simulink model "RegulatedBuckConverter"  (R2021b)
settings: Solver=ode23tb  StartTime=0.0  StopTime=0.5  RelTol=1e-4  EnableMultiTasking=on
PreLoadFcn:
  | Ts=10e-6;
InitFcn:
  | Ts=10e-6;
libraries: spsGroundLib x3, spsDCVoltageSourceLib x2, spsBuckConverterLib x1, spsDCMachineLib x1, spsFirstOrderFilterLib x1, spsSeriesRLCBranchLib x1, spsMeanLib x1, spsVoltageMeasurementLib x1, spspowerguiLib x1
settings Model: Creator=The MathWorks, Inc.  LastModifiedBy=francescobazzani
settings SolverCC: AlgebraicLoopSolver=TrustRegion  SolverResetMethod=Robust
settings DataIOCC: SaveFormat=StructureWithTime  SaveOutput=off  SignalLogging=off  DSMLogging=off  VisualizeSimOutput=off  SaveTime=off  ReturnWorkspaceOutputs=off
settings OptimizationCC: LifeSpan=inf
settings DebuggingCC: UnconnectedInputMsg=none  UnconnectedOutputMsg=none  UnconnectedLineMsg=none  AllowSymbolicDim=off  SFUnexpectedBacktrackingDiag=warning  SFNoUnconditionalDefaultTransitionDiag=warning  SFExecutionAtInitializationDiag=none  SFMachineParentedDataDiag=warning  ArithmeticOperatorsInVariantConditions=warning
settings ModelReferenceCC: PropagateSignalLabelsOutOfModel=off
settings SFSimCC: SimUseLocalCustomCode=off  CustomCodeUndefinedFunction=UseInterfaceOnly
settings RTWCC: RTWUseLocalCustomCode=off
settings CodeAppCC: StateflowObjectComments=on
settings GRTTargetCC: TargetLangStandard=C89/C90 (ANSI)
settings ConfigComp: CovMetricSettings=dw  CovSaveCumulativeToWorkspaceVar=on  CovSaveSingleToWorkspaceVar=on  CovExternalEMLEnable=off
settings SimscapeCC: SimscapeNormalizeSystem=off  SimscapeNominalValues={1, 'bar'; 1, 'cm^3/s'; 1, 'bar*kg/s'; 1, 'kJ/kg'; 1, 'kW'; }

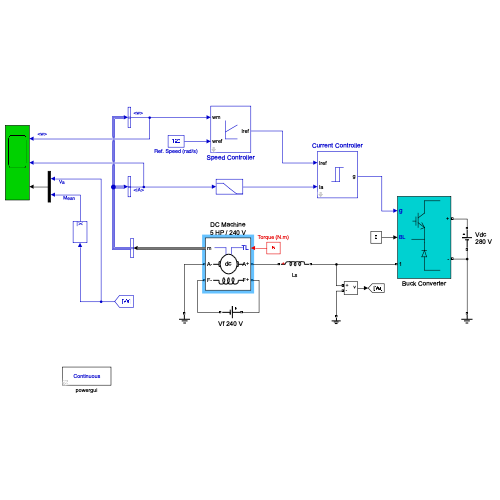
[thumbnail: Simulink's stored preview of the top-level diagram]
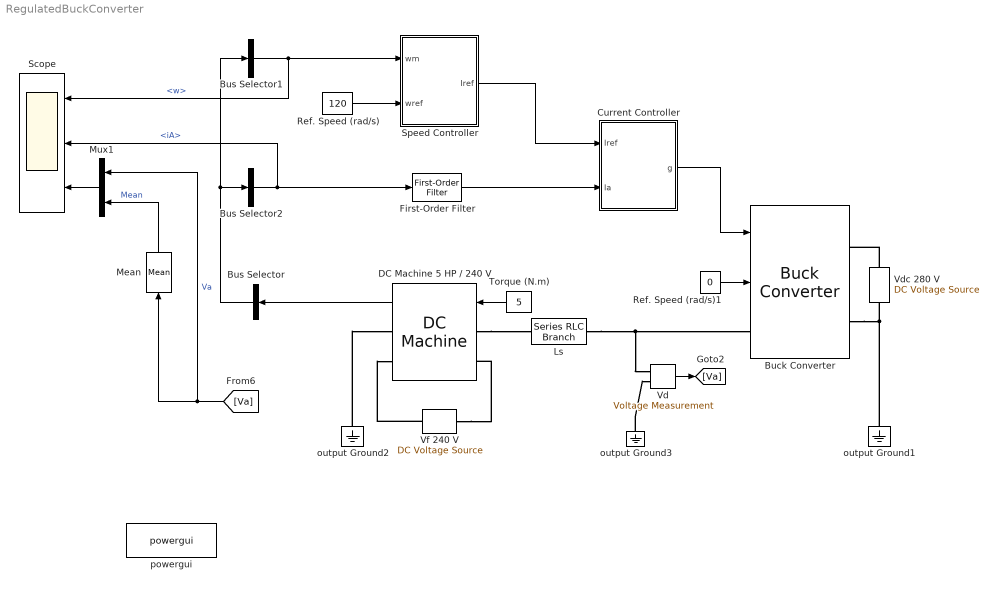
== system RegulatedBuckConverter ==
  Buck Converter : spsBuckConverterLib/Buck Converter  ModelType=Switching devices  Ron=1e-3  Rs=1e6  Cs=inf  Vforward=[0,0]  Ron_Diode=1e-3  Rs_Diode=1e6  Cs_Diode=inf  Vf_Diode=1e-3  Rs_CurrentSource=inf
      settings: SourceProductBaseCode=PS
  Bus Selector : BusSelector  OutputSignals=w,iA  OutputAsBus=on
  Bus Selector1 : BusSelector  OutputSignals=w
  Bus Selector2 : BusSelector  OutputSignals=iA
  Current Controller : Subsystem  mask{h=2}
      mask prompts: h "Hysteresis band (A)"
      mask help: Hysteresis Current Controller
      mask Display: plot(0,0,100,100,[45,45],[35,65],[55,55],[35,65],[45,65],[65,65],[35,55],[35,35])
  DC Machine 5 HP / 240 V : spsDCMachineLib/DC Machine  PresetModel=No  MechanicalLoad=Torque TL  FieldType=Wound  ShowDetailedParameters=on  MeasurementBus=on  RLa="[ 0.5  0.01]"  RLf="[ 240  120]"  Laf=1.23  MachineConstant=Torque constant (N.m/A)  Ke=1.8  Kt=1.8  J=0.05  Bm=0.02  Tf=0  w0=0  Ifinit=1  TsPowergui=0  TsBlock=-1
  First-Order Filter : spsFirstOrderFilterLib/First-Order Filter  FilterType=Lowpass  Tc=10e-6  Ts=0  Initialize=off  Vac_Init=[0, 0, 60]  Vdc_Init=0  PlotResponse=off  FreqRange="[0,  200,  1]"
  Ls : spsSeriesRLCBranchLib/Series RLC Branch  LConnTagsString=__new0  RConnTagsString=__new0  BranchType=L  Resistance=0.01  Inductance=10e-3  SetiL0=off  InitialCurrent=30  Capacitance=[]  Setx0=off  InitialVoltage=0  Measurements=None
  Mean : spsMeanLib/Mean  Freq=60  Vinit=0  Ts=0
  Mux1 : Mux  Inputs=2
  Ref. Speed (rad/s) : Constant  Value=120
  Ref. Speed (rad/s)1 : Constant  Value=0
  Scope : Scope  NumInputPorts=3
  Speed Controller : Subsystem  mask(PI controller){Kp=1.6, Ki=16, Ilim=30}
      mask prompts: Kp "Proportional gain (Kp)"; Ki "Integral gain (Ki)"; Ilim "Current limit (A)"
      mask help: Proportional-Integral Speed Controller
      mask Display: plot(0,0,100,100,[35,35,65],[70,30,30],[35,65],[45,60])
  Torque (N.m) : Constant  Value=5
  Vd : spsVoltageMeasurementLib/Voltage Measurement  Tag=PoWeRsYsTeMmEaSuReMeNt  PhasorSimulation=off  OutputType=Complex  PSBequivalent=0
  "Vdc 280 V " : spsDCVoltageSourceLib/DC Voltage Source  Description=source block  Amplitude=280  Measurements=None
      settings: AttributesFormatString=\n
  Vf 240 V : spsDCVoltageSourceLib/DC Voltage Source  Description=source block  Amplitude=240  Measurements=None
      settings: AttributesFormatString=\n
  output Ground1 : spsGroundLib/Ground  LConnTagsString=a
  output Ground2 : spsGroundLib/Ground  LConnTagsString=a
  output Ground3 : spsGroundLib/Ground  LConnTagsString=a
  powergui : spspowerguiLib/powergui  Priority=1  SimulationMode=Continuous  SampleTime=10e-6  frequency=60  Iterations=50  frequencyindice=0  Pbase=100e6  ErrMax=0.0001  UnitsV=kV  UnitsW=MW  buscounter=0  FunctionMessages=off  echomessages=off  EnableUseOfTLC=off  CurrentSourceSwitches=off  DisableSnubberDevices=on  DisableRonSwitches=off  DisableVfSwitches=on  DisplayEquations=off  AutomaticDiscreteSolvers=off  SolverType=Tustin/Backward Euler (TBE)  Interpol=off  ExternalGateDelay=off  methode=off  Ts=10  x0status=blocks  SPID=on  SwTol=0  HookPort=off  NonlinearTolerance=1e-4  nMaxIteration=100  ContinueOnMaxIteration=off  RestoreLinks=warning  ResistiveCurrentMeasurement=off  Frange=[0:2:500]  Ylog=off  Xlog=on  ShowGrid=off  save=off  variable=ZData  structure=ScopeData1  ZoomFFT=off  StartTime=0.04  cycles=1  DisplayStyle=1  fundamental=60  FreqAxis=on  MaxFrequency=1200  frequencyindicesteady=1  RmsSteady=1  display=off
  wires:
  Vd/1 -> [Va]
  Mean/1 -> Mux1/2  "Mean"
  Mux1/1 -> Scope/3
  Torque (N.m)/1 -> DC Machine 5 HP / 240 V/1
  Current Controller/1(g) -> Buck Converter/1
  DC Machine 5 HP / 240 V/1 -> Bus Selector/1
  Ref. Speed (rad/s)1/1 -> Buck Converter/2
  [Va] -> Mean/1, Mux1/1  "Va"
  Bus Selector/1 -> Bus Selector1/1, Bus Selector2/1
  Bus Selector1/1 -> Scope/1, Speed Controller/1(wm)  "<w>"
  Ref. Speed (rad/s)/1 -> Speed Controller/2(wref)
  Bus Selector2/1 -> Scope/2, First-Order Filter/1  "<iA>"
  Speed Controller/1(Iref) -> Current Controller/1(Iref)
  First-Order Filter/1 -> Current Controller/2(Ia)
  connections:
  output Ground1/LConn1 -- Buck Converter/RConn2 -- "Vdc 280 V "/LConn1
  "Vdc 280 V "/RConn1 -- Buck Converter/RConn1
  Ls/RConn1 -- Buck Converter/LConn1 -- Vd/LConn1
  Vf 240 V/RConn1 -- DC Machine 5 HP / 240 V/LConn2
  Vf 240 V/LConn1 -- DC Machine 5 HP / 240 V/RConn2
  DC Machine 5 HP / 240 V/LConn1 -- Ls/LConn1
  output Ground2/LConn1 -- DC Machine 5 HP / 240 V/RConn1
  output Ground3/LConn1 -- Vd/LConn2

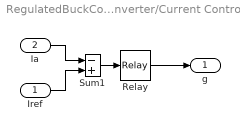
== system RegulatedBuckConverter/Current Controller ==
  Iref : Inport
  Ia : Inport  Port=2
  Relay : Relay  OnSwitchValue=h/2  OffSwitchValue=-h/2
  Sum1 : Sum  Inputs=-+  InputSameDT=on  SaturateOnIntegerOverflow=on  OutDataTypeStr=Inherit: Same as first input
  g : Outport  InitialOutput=0  VectorParamsAs1DForOutWhenUnconnected=off
  wires:
  Iref/1 -> Sum1/2
  Ia/1 -> Sum1/1
  Relay/1 -> g/1
  Sum1/1 -> Relay/1

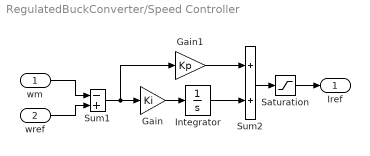
== system RegulatedBuckConverter/Speed Controller ==
  wm : Inport
  wref : Inport  Port=2
  Gain : Gain  Gain=Ki  SaturateOnIntegerOverflow=on  OutDataTypeStr=Inherit: Same as input  ParamDataTypeStr=Inherit: Same as input
  Gain1 : Gain  Gain=Kp  SaturateOnIntegerOverflow=on  OutDataTypeStr=Inherit: Same as input  ParamDataTypeStr=Inherit: Same as input
  Integrator : Integrator  LimitOutput=on  UpperSaturationLimit=Ilim  LowerSaturationLimit=-Ilim
  Saturation : Saturate  UpperLimit=Ilim  LowerLimit=-Ilim
  Sum1 : Sum  Inputs=-+  InputSameDT=on  SaturateOnIntegerOverflow=on  OutDataTypeStr=Inherit: Same as first input
  Sum2 : Sum  InputSameDT=on  SaturateOnIntegerOverflow=on  OutDataTypeStr=Inherit: Same as first input
  Iref : Outport  InitialOutput=0  VectorParamsAs1DForOutWhenUnconnected=off
  wires:
  Gain1/1 -> Sum2/1
  Gain/1 -> Integrator/1
  Sum1/1 -> Gain/1, Gain1/1
  wm/1 -> Sum1/1
  wref/1 -> Sum1/2
  Integrator/1 -> Sum2/2
  Sum2/1 -> Saturation/1
  Saturation/1 -> Iref/1
